simulink model "Applied_Dynamics"  (R2021a)
settings: Solver=VariableStepAuto  StartTime=0.0  StopTime=10.0  RelTol=1e-3
undefined symbols (not defined in the file): a1, a2, b
settings Model: Creator=ragnarzone  LastModifiedBy=ragnarzone

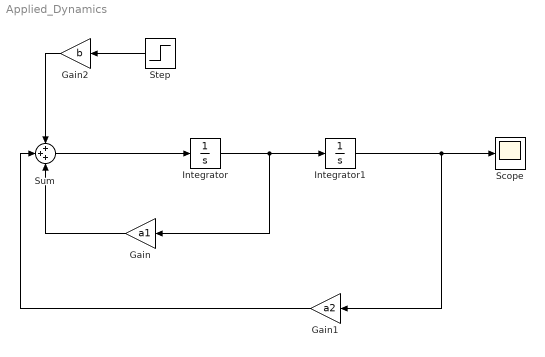
== system Applied_Dynamics ==
  Gain : Gain  Gain=a1
  Gain1 : Gain  Gain=a2
  Gain2 : Gain  Gain=b
  Integrator : Integrator
  Integrator1 : Integrator
  Scope : Scope
  Step : Step  SampleTime=0
  Sum : Sum  Inputs=+++
  wires:
  Integrator/1 -> Gain/1, Integrator1/1
  Sum/1 -> Integrator/1
  Gain1/1 -> Sum/2
  Step/1 -> Gain2/1
  Gain/1 -> Sum/3
  Integrator1/1 -> Scope/1, Gain1/1
  Gain2/1 -> Sum/1
